simulink model "Waage_simulink"  (R2025a)
settings: Solver=VariableStepAuto  StartTime=0.0  StopTime=3  FixedStep=0.001  RelTol=1e-3
undefined symbols (not defined in the file): C, g, k, Kd, Kf, mw, R_L, U_max
libraries: slpidlib x1
settings Model: Creator=bme22w09  LastModifiedBy=zeyadsaadaddin
settings OptimizationCC: ReuseModelBlockBuffer=off
settings RTWCC: GPUComputeCapability=3.5

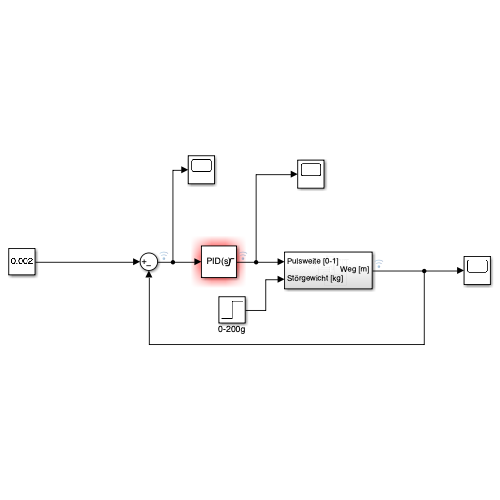
[thumbnail: Simulink's stored preview of the top-level diagram]
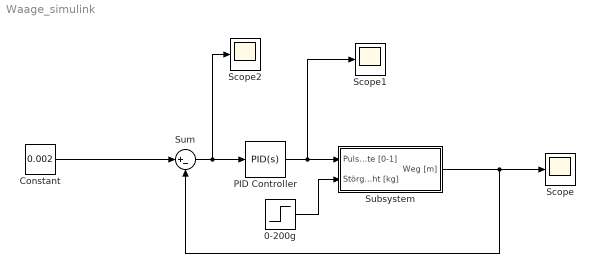
== system Waage_simulink ==
  0-200g : Step  Time=2  After=0.2  SampleTime=0
  Constant : Constant  Value=0.002
  PID Controller : slpidlib/PID Controller  Controller=PID  Form=Parallel  TimeDomain=Continuous-time  UseExternalTs=off  SampleTime=-1  IntegratorMethod=Forward Euler  FilterMethod=Forward Euler  ControllerParametersSource=internal  P=C.Kp  I=C.Ki  UseKiTs=off  D=C.Kd  UseExternalDerivativeSource=off  N=100  UseFilter=on  TunerSelectOption=Transfer Function Based (PID Tuner App)  InitialConditionSource=internal  InitialConditionForIntegrator=0  InitialConditionForFilter=0  DifferentiatorICPrevScaledInput=0  ExternalReset=none  TrackingMode=off  Kt=1  LimitOutput=on  SatLimitsSource=internal  UpperSaturationLimit=1  LowerSaturationLimit=0  LinearizeAsGain=on  AntiWindupMode=clamping  Kb=1  LimitIntegrator=off  UpperIntegratorSaturationLimit=inf  LowerIntegratorSaturationLimit=-inf  POutMin=[]  POutMax=[]  IOutMin=[]  IOutMax=[]  DOutMin=[]  DOutMax=[]  NOutMin=[]  NOutMax=[]  SumOutMin=[]  SumOutMax=[]  SaturationOutMin=[]  SaturationOutMax=[]  PParamMin=[]  PParamMax=[]  IParamMin=[]  IParamMax=[]  DParamMin=[]  DParamMax=[]  NParamMin=[]  NParamMax=[]  KbParamMin=[]  KbParamMax=[]  KtParamMin=[]  KtParamMax=[]  KbOutMin=[]  KbOutMax=[]  KtOutMin=[]  KtOutMax=[]  IntegratorOutMin=[]  IntegratorOutMax=[]  FilterOutMin=[]  FilterOutMax=[]  SumI1OutMin=[]  SumI1OutMax=[]  SumI2OutMin=[]  SumI2OutMax=[]  SumI3OutMin=[]  SumI3OutMax=[]  SumI4OutMin=[]  SumI4OutMax=[]  SumDOutMin=[]  SumDOutMax=[]  DifferentiatorOutMin=[]  DifferentiatorOutMax=[]  FilterDiffOutCoefMin=[]  FilterDiffOutCoefMax=[]  ReciprocalOutMin=[]  ReciprocalOutMax=[]  SumDenOutMin=[]  SumDenOutMax=[]  SumNumOutMin=[]  SumNumOutMax=[]  DivideOutMin=[]  DivideOutMax=[]  UdiffTsProdOutMin=[]  UdiffTsProdOutMax=[]  NTsProdOutMin=[]  NTsProdOutMax=[]  UintegralTsProdOutMin=[]  UintegralTsProdOutMax=[]  UngainTsProdOutMin=[]  UngainTsProdOutMax=[]  ClampingZeroOutDataTypeStr=Inherit: Inherit via back propagation  ClampingZeroOutMin=[]  ClampingZeroOutMax=[]  FilterDenConstantOutDataTypeStr=Inherit: Inherit via back propagation  FilterDenConstantOutMin=[]  FilterDenConstantOutMax=[]  PCopyOutDataTypeStr=Inherit: Inherit via back propagation  PCopyOutMin=[]  PCopyOutMax=[]  NCopyOutDataTypeStr=Inherit: Inherit via back propagation  NCopyOutMin=[]  NCopyOutMax=[]  IntegratorContinuousStateAttributes=''  IntegratorStateMustResolveToSignalObject=off  IntegratorRTWStateStorageClass=Auto  FilterContinuousStateAttributes=''  FilterStateMustResolveToSignalObject=off  FilterRTWStateStorageClass=Auto  ParallelPVariant=InternalParameters  IdealPVariant=Disabled  IVariant=InternalParameters  DVariant=InternalParameters  IntegratorVariant=Continuous  SatVariant=Enabled  AWVariant=ContClampingParallel  PCopyVariant=Disabled  TRVariant=Disabled  FdbkBlocksVariant=Forward  IdealPFdbkVariant=Disabled  SatFdbkVariant=Disabled  DerivativeFilterVariant=ContFilter  NVariant=InternalParameters  NCopyVariant=Disabled  FilterICVariant=InternalICsFilter  IntegratorICVariant=InternalICs  ExternalResetVariant=Disabled  TRSumVariant=Passthrough  SumFdbkVariant=Disabled  SumVariant=Sum_PID  TsampFilterVariant=InternalTs  TsampNgainVariant=Passthrough  TsampIntegralVariant=Disabled_SignalSpec  ExternalSaturationOutDataTypeStr=Inherit: Same as second input  DerivativeSourceVariant=ErrorSignal  PreIntVariant=InternalPreInt
  Scope : Scope
      settings: ActiveDisplayYMinimum=-0.00026  ActiveDisplayYMaximum=0.00236
  Scope1 : Scope
      settings: ActiveDisplayYMinimum=-0.00959  ActiveDisplayYMaximum=0.23924
  Scope2 : Scope
      settings: ActiveDisplayYMinimum=-0.00036  ActiveDisplayYMaximum=0.00226  DataLoggingVariableName=ScopeData2
  Subsystem : Subsystem
  Sum : Sum  Inputs=|+-
  wires:
  Subsystem/1(Weg [m]) -> Sum/2, Scope/1
  Constant/1 -> Sum/1
  Sum/1 -> Scope2/1, PID Controller/1
  0-200g/1 -> Subsystem/2(Störgewicht [kg])
  PID Controller/1 -> Scope1/1, Subsystem/1(Pulsweite [0-1])

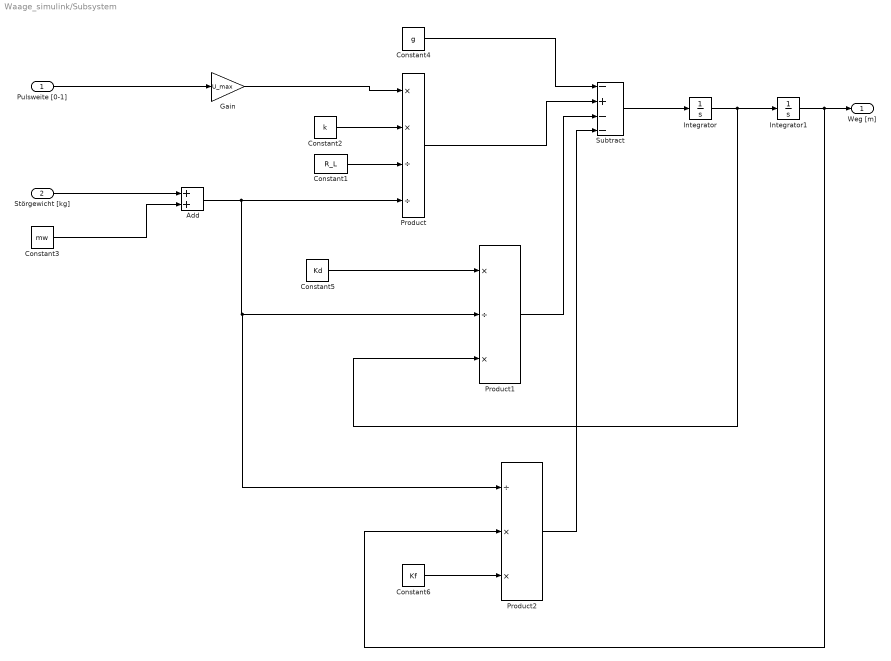
== system Waage_simulink/Subsystem ==
  Pulsweite [0-1] : Inport
  Störgewicht [kg] : Inport  Port=2
  Add : Sum
  Constant1 : Constant  Value=R_L
  Constant2 : Constant  Value=k
  Constant3 : Constant  Value=mw
  Constant4 : Constant  Value=g
  Constant5 : Constant  Value=Kd
  Constant6 : Constant  Value=Kf
  Gain : Gain  Gain=U_max
  Integrator : Integrator
  Integrator1 : Integrator  LimitOutput=on  UpperSaturationLimit=0.004  LowerSaturationLimit=0
  Product : Product  Inputs=**//
  Product1 : Product  Inputs=*/*
  Product2 : Product  Inputs=/**
  Subtract : Sum  Inputs=-+--
  Weg [m] : Outport
  wires:
  Product/1 -> Subtract/2
  Störgewicht [kg]/1 -> Add/1
  Constant3/1 -> Add/2
  Constant1/1 -> Product/3
  Constant2/1 -> Product/2
  Constant4/1 -> Subtract/1
  Add/1 -> Product2/1, Product1/2, Product/4
  Subtract/1 -> Integrator/1
  Integrator/1 -> Product1/3, Integrator1/1
  Integrator1/1 -> Product2/2, Weg [m]/1
  Product1/1 -> Subtract/3
  Constant5/1 -> Product1/1
  Pulsweite [0-1]/1 -> Gain/1
  Gain/1 -> Product/1
  Constant6/1 -> Product2/3
  Product2/1 -> Subtract/4
